simulink model "Digital_PID_on_Simulink"  (R2025b)
settings: Solver=FixedStepAuto  StartTime=0.0  StopTime=inf  RelTol=1e-3  EnableMultiTasking=on
undefined symbols (not defined in the file): DiscIntNeverNeededParam
libraries: arduinolib x4, simulink x1, arduinoavrlib x1
settings Model: ExtModeTrigDuration=2  Creator=MSI  LastModifiedBy=MSI
settings SolverCC: AutoInsertRateTranBlk=on
settings OptimizationCC: EnhancedBackFolding=on  PassReuseOutputArgsAs=Individual arguments  ZeroExternalMemoryAtStartup=off  ZeroInternalMemoryAtStartup=off  MaxStackSize=64  OptimizeBlockOrder=speed  DifferentSizesBufferReuse=on  OptimizationCustomize=off  EfficientTunableParamExpr=on
settings DebuggingCC: ParameterTunabilityLossMsg=error
settings HardwareCC: ProdBitPerInt=16.0  ProdBitPerPointer=16.0  ProdBitPerSizeT=16.0  ProdBitPerPtrDiffT=16.0  ProdLargestAtomicFloat=None  ProdWordSize=8.0  ProdHWDeviceType=Atmel->AVR
settings SFSimCC: MATLABDynamicMemAlloc=off
settings RTWCC: SystemTargetFile=ert.tlc  HardwareBoard=Arduino Uno  TemplateMakefile=ert_default_tmf  Toolchain=Arduino AVR  BuildConfiguration=Faster Runs  Description=Embedded Coder
settings CodeAppCC: ForceParamTrailComments=on  IgnoreCustomStorageClasses=off  OperatorAnnotations=on  SimulinkDataObjDesc=on  SFDataObjDesc=on  InsertBlockDesc=on
settings ERTTargetCC: ExtModeTransport=3.0  ExtModeStaticAlloc=on  ExtModeAutomaticAllocSize=off  ExtModeStaticAllocSize=250.0  ExtModeMexFile=ext_xcp  ExtModeIntrfLevel=Level2 - Open  InlinedParameterPlacement=Hierarchical  SupportContinuousTime=on  SupportVariableSizeSignals=on

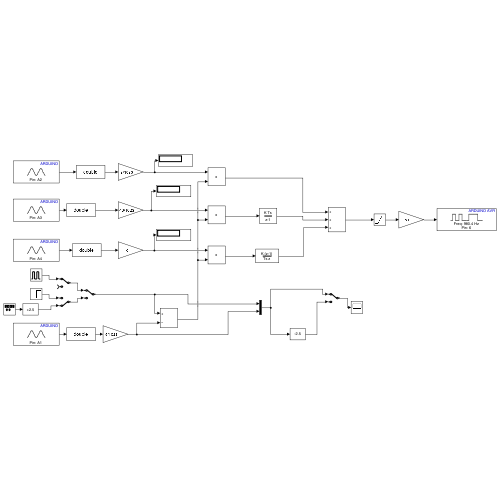
[thumbnail: Simulink's stored preview of the top-level diagram]
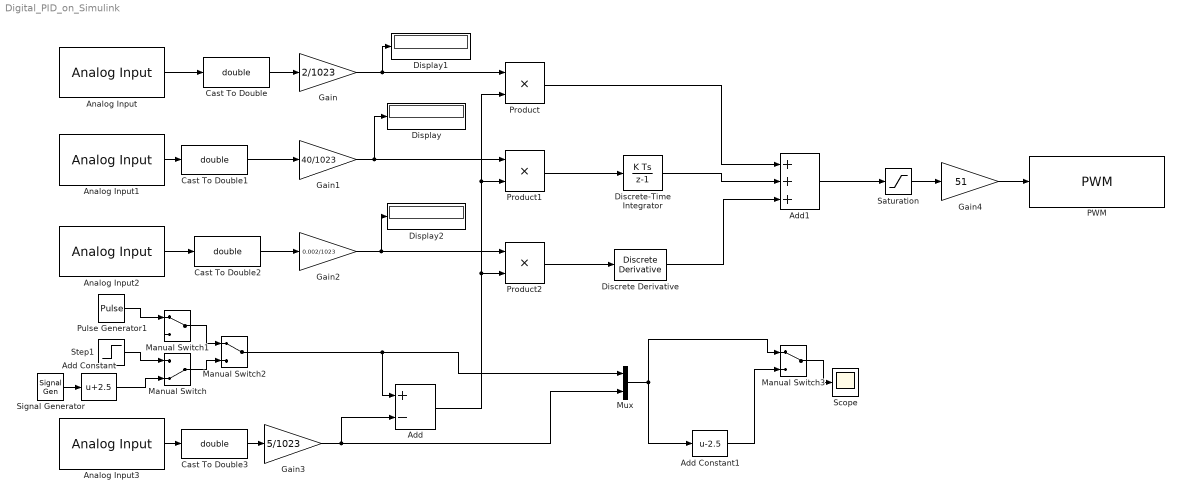
== system Digital_PID_on_Simulink ==
  Add : Sum  Inputs=+-
  Add Constant : Bias  Bias=2.5  SaturateOnIntegerOverflow=off
  Add Constant1 : Bias  Bias=-2.5  SaturateOnIntegerOverflow=off
  Add1 : Sum  Inputs=+++
  Analog Input : arduinolib/Analog Input  pinNumber=2  ReadResultsOnly=off  ConversionTriggerSource=Software  ExternalTriggerType=uint32( 0 )  OutputDataType=uint16  EnableConversionCompleteNotify=off  EnableOuputStatus=off  SampleTime=0.01  blockPlatform=arduino
  Analog Input1 : arduinolib/Analog Input  pinNumber=3  ReadResultsOnly=off  ConversionTriggerSource=Software  ExternalTriggerType=uint32( 0 )  OutputDataType=uint16  EnableConversionCompleteNotify=off  EnableOuputStatus=off  SampleTime=0.01  blockPlatform=arduino
  Analog Input2 : arduinolib/Analog Input  pinNumber=4  ReadResultsOnly=off  ConversionTriggerSource=Software  ExternalTriggerType=uint32( 0 )  OutputDataType=uint16  EnableConversionCompleteNotify=off  EnableOuputStatus=off  SampleTime=0.01  blockPlatform=arduino
  Analog Input3 : arduinolib/Analog Input  pinNumber=1  ReadResultsOnly=off  ConversionTriggerSource=Software  ExternalTriggerType=uint32( 0 )  OutputDataType=uint16  EnableConversionCompleteNotify=off  EnableOuputStatus=off  SampleTime=0.01  blockPlatform=arduino
  Cast To Double{,1..3} (4 alike) : DataTypeConversion  OutDataTypeStr=double  SaturateOnIntegerOverflow=off  RndMeth=Floor
  Discrete Derivative : simulink/Discrete/Discrete Derivative  gainval=1.0  ICPrevScaledInput=0.0  OutMin=[]  OutMax=[]  OutDataType=fixdt(1, 16)  OutScaling=2^-10  DoSatur=off
  Discrete-Time Integrator : DiscreteIntegrator  SampleTime=0.01  ICPrevOutput=DiscIntNeverNeededParam  ICPrevScaledInput=DiscIntNeverNeededParam
  Display : Display
  Display1 : Display
  Display2 : Display
  Gain : Gain  Gain=2/1023
  Gain1 : Gain  Gain=40/1023
  Gain2 : Gain  Gain=0.002/1023
  Gain3 : Gain  Gain=5/1023
  Gain4 : Gain  Gain=51
  Manual Switch : ManualSwitch  CurrentSetting=0
  Manual Switch1 : ManualSwitch
  Manual Switch2 : ManualSwitch
  Manual Switch3 : ManualSwitch
  Mux : Mux  Inputs=2
  PWM : arduinoavrlib/PWM  pinNumber=6  desiredFrequency=980.4  achievableFrequency=980.4  EnableCompareMatchInterrupt=off  EnableOverflowInterrupt=off
  Product : Product
  Product1 : Product
  Product2 : Product
  Pulse Generator1 : DiscretePulseGenerator  PulseType=Time based  Amplitude=5  Period=4  PulseWidth=50
  Saturation : Saturate  UpperLimit=5  LowerLimit=0
  Scope : Scope
      settings: ActiveDisplayYMinimum=-0.62499999999999989  ActiveDisplayYMaximum=5.625
  Signal Generator : SignalGenerator  Amplitude=2.5  Frequency=4  Units=rad/sec
  Step1 : Step  After=5  SampleTime=0
  wires:
  Analog Input/1 -> Cast To Double/1
  Analog Input1/1 -> Cast To Double1/1
  Analog Input2/1 -> Cast To Double2/1
  Analog Input3/1 -> Cast To Double3/1
  Gain3/1 -> Mux/2, Add/2
  Gain/1 -> Display1/1, Product/1
  Gain1/1 -> Display/1, Product1/1
  Gain2/1 -> Display2/1, Product2/1
  Add/1 -> Product2/2, Product1/2, Product/2
  Product1/1 -> Discrete-Time Integrator/1
  Product2/1 -> Discrete Derivative/1
  Product/1 -> Add1/1
  Discrete-Time Integrator/1 -> Add1/2
  Discrete Derivative/1 -> Add1/3
  Add1/1 -> Saturation/1
  Saturation/1 -> Gain4/1
  Gain4/1 -> PWM/1
  Cast To Double/1 -> Gain/1
  Cast To Double1/1 -> Gain1/1
  Cast To Double2/1 -> Gain2/1
  Cast To Double3/1 -> Gain3/1
  Step1/1 -> Manual Switch/1
  Signal Generator/1 -> Add Constant/1
  Pulse Generator1/1 -> Manual Switch1/1
  Manual Switch1/1 -> Manual Switch2/1
  Manual Switch/1 -> Manual Switch2/2
  Manual Switch2/1 -> Add/1, Mux/1
  Add Constant/1 -> Manual Switch/2
  Mux/1 -> Manual Switch3/1, Add Constant1/1
  Manual Switch3/1 -> Scope/1
  Add Constant1/1 -> Manual Switch3/2
